simulink model "state_space"  (R2015a)
settings: Solver=ode4  StartTime=0.0  StopTime=5  FixedStep=0.01  RelTol=1e-3
values from neighbouring files (symbols this model uses):
  A = [ ... (first row only)    [ex_expm.m]    (also in ex_residue.m; mimo_test.m; plant.m = [0 1)
  B = [ ... (first row only)    [mimo_test.m]    (also in plant.m = [0 1]')
  C = [ ... (first row only)    [mimo_test.m]    (also in plant.m = [1 0])
  D = [ ... (first row only)    [mimo_test.m]    (also in plant.m = 0)
  x0 = [1 0]'    [ex_expm.m]    (also in ex_residue.m; mimo_test.m = [1 0 -1 0]'; plant.m)
settings Model: Creator=shohei  LastModifiedBy=shohei

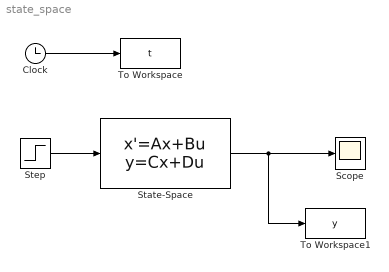
== system state_space ==
  Clock : Clock
  Scope : Scope
  State-Space : StateSpace  A=A  B=B  C=C  D=D  X0=x0
  Step : Step  SampleTime=0
  To Workspace : ToWorkspace  VariableName=t  SaveFormat=Timeseries  SampleTime=-1
  To Workspace1 : ToWorkspace  VariableName=y  SaveFormat=Timeseries  SampleTime=-1
  wires:
  Clock/1 -> To Workspace/1
  Step/1 -> State-Space/1
  State-Space/1 -> To Workspace1/1, Scope/1
